simulink library "WDB2THB"  (R2018b)
settings: Solver=ode45  StartTime=0.0  StopTime=10.0  RelTol=1e-3  EnableMultiTasking=on
undefined symbols (not defined in the file): FluidMix, Pressure, Temperature
libraries: carnot x2
settings Model: Creator=lena.frank  LastModifiedBy=drhf
settings DataIOCC: LimitDataPoints=on  SaveFormat=Array  SignalLoggingSaveFormat=ModelDataLogs
settings OptimizationCC: ExpressionDepthLimit=2147483647  LifeSpan=inf
settings DebuggingCC: UnderspecifiedInitializationDetection=Classic  MergeDetectMultiDrivingBlocksExec=none  SolverPrmCheckMsg=warning  FcnCallInpInsideContextMsg=warning  StateNameClashWarn=warning  SFUnexpectedBacktrackingDiag=warning  SFNoUnconditionalDefaultTransitionDiag=warning  SFExecutionAtInitializationDiag=none
settings HardwareCC: ProdBitPerPointer=32  ProdBitPerSizeT=32  ProdBitPerPtrDiffT=32  ProdLargestAtomicFloat=None  ProdIntDivRoundTo=Undefined  ProdEndianess=Unspecified  ProdWordSize=32  ProdHWDeviceType=32-bit Generic
settings ModelReferenceCC: PropagateSignalLabelsOutOfModel=off
settings SFSimCC: SimUseLocalCustomCode=off
settings RTWCC: RTWUseLocalCustomCode=off
settings CodeAppCC: StateflowObjectComments=on
settings GRTTargetCC: TargetLangStandard=C89/C90 (ANSI)  GeneratePreprocessorConditionals=Disable all  CombineOutputUpdateFcns=off  GRTInterface=on
settings ConfigComp: CovMetricSettings=dw  CovHtmlReporting=on  CovSaveCumulativeToWorkspaceVar=on  CovSaveSingleToWorkspaceVar=on  CovExternalEMLEnable=off

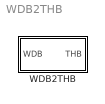
== system WDB2THB ==
  WDB2THB : Subsystem  mask(Weather Data Bus to Thermo Hydraulic Bus){dia=0.2}
      mask prompts: dia "diameter [m]"
      mask help: Transfers the incoming weather data to an air flow in the thermo-hydraulic vector THV. All properties are set to ambient conditions (temperature, pressure, humidity).
      mask init:
      | dia = max(dia, 0.001);
      mask Help: web(fullfile(path_carnot('help'),'WDB2THB.html'),'-helpbrowser')

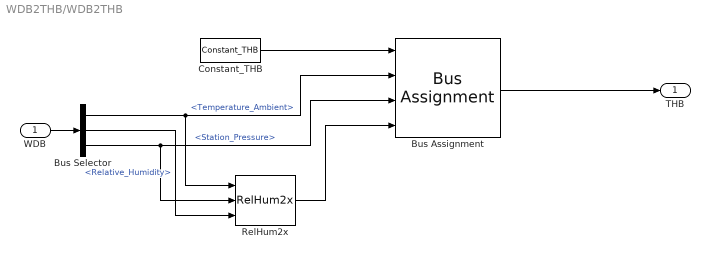
== system WDB2THB/WDB2THB ==
  WDB : Inport
  Bus Assignment : BusAssignment  AssignedSignals=Temperature,Pressure,FluidMix
  Bus Selector : BusSelector  OutputSignals=Temperature_Ambient,Relative_Humidity,Station_Pressure
  Constant_THB : carnot/Source/Simple/Constant_THB  t=10  mdot=0  p=1e5  mID=No Pressure Drop  fluid=Air  mix=0  dia=dia  hgt=0
      settings: SourceProductName=Carnot
  RelHum2x : carnot/Basic/Material_Properties/RelHum2x
      settings: SourceProductName=Carnot
  THB : Outport
  wires:
  WDB/1 -> Bus Selector/1
  Constant_THB/1 -> Bus Assignment/1
  Bus Assignment/1 -> THB/1
  Bus Selector/1 -> RelHum2x/1, Bus Assignment/2  "<Temperature_Ambient>"
  Bus Selector/2 -> RelHum2x/3  "<Relative_Humidity>"
  Bus Selector/3 -> RelHum2x/2, Bus Assignment/3  "<Station_Pressure>"
  RelHum2x/1 -> Bus Assignment/4
